simulink model "AdvancedRobotics_PA2_Exercise3"  (R2022a)
settings: Solver=VariableStepAuto  StartTime=0.0  StopTime=10  RelTol=1e-3
values from neighbouring files (symbols this model uses):
  C = CM+CL/n^2    (= 0.0001425)    [AdvancedRobotics_PA2_Exercise3.m]    (also in ControlSystem_transfer_function_ztransform.m = [0 1]; MechDesign_Exercise3_Assessment1.m = k1-(k2+1)*cos(theta_2/180*pi)+k3; PIDTurner.m = pid(Kp,0,Kd); TransferfunctionStateSpace.m = [1 0])
  g = sind(TH2).*sind(TH4) - cosd(TH2).*cosd(TH3).*cosd(TH4)    [AdvancedRobotics_PA2_Exercise2_Group.m]    (also in AdvancedRobotics_PA2_Exercise3.m = 386.1; DigitalFundamental_Lab1_Group.m = 9.8; DigitalFundamental_individual_project_milestone.m = oz*28.3495)
  J = JM+JL/n^2    (= 0.008465)    [AdvancedRobotics_PA2_Exercise3.m]    (also in TransferfunctionStateSpace.m = 0.01)
  Ka = 12    [AdvancedRobotics_PA2_Exercise3.m]
  Kb = 0.00867    [AdvancedRobotics_PA2_Exercise3.m]
  Ke = 1    [AdvancedRobotics_PA2_Exercise3.m]
  KM = 4.375    [AdvancedRobotics_PA2_Exercise3.m]
  L = 0.278    [AdvancedRobotics_PA2_Exercise1_Group.m]    (also in AdvancedRobotics_PA2_Exercise3.m = 0.0006; TransferfunctionStateSpace.m = 0.5)
  l = 6.4    [AdvancedRobotics_PA2_Exercise3.m]
  m = 200    [AdvancedRobotics_PA2_Exercise3.m]    (also in ControlSystem_transfer_function_ztransform.m = 1; DigitalFundamental_individual_project_milestone.m = ft*0.3048)
  n = 200    [AdvancedRobotics_PA2_Exercise3.m]
  R = 1.4    [AdvancedRobotics_PA2_Exercise3.m]    (also in TransferfunctionStateSpace.m = 1)
libraries: simulink x4, slpidlib x2
settings Model: Creator=Thanh  LastModifiedBy=Thanh

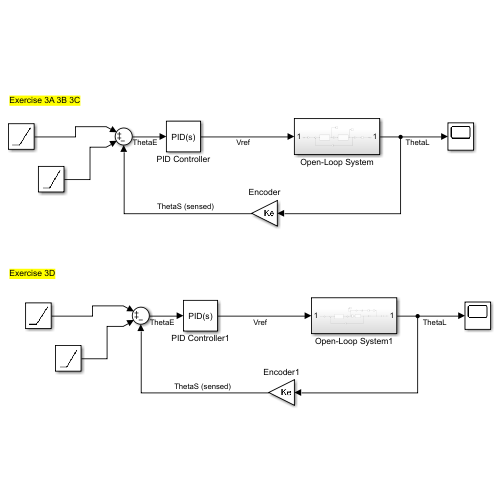
[thumbnail: Simulink's stored preview of the top-level diagram]
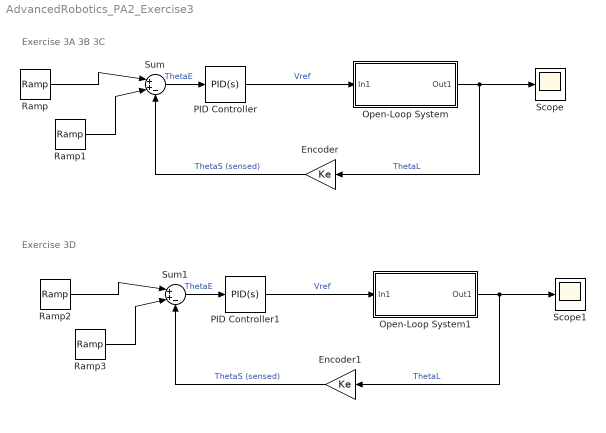
== system AdvancedRobotics_PA2_Exercise3 ==
  note: Exercise 3D
  note: Exercise 3A 3B 3C
  Encoder : Gain  Gain=Ke
  Encoder1 : Gain  Gain=Ke
  Open-Loop System : Subsystem
  Open-Loop System1 : Subsystem
  PID Controller : slpidlib/PID Controller  Controller=PID  Form=Parallel  TimeDomain=Continuous-time  UseExternalTs=off  SampleTime=-1  IntegratorMethod=Forward Euler  FilterMethod=Forward Euler  ControllerParametersSource=internal  P=3.93142383179375  I=1.32077543733285  UseKiTs=off  D=2.60010998792399  N=6581.10544930307  UseFilter=on  TunerSelectOption=Transfer Function Based (PID Tuner App)  InitialConditionSource=internal  InitialConditionForIntegrator=0  InitialConditionForFilter=0  DifferentiatorICPrevScaledInput=0  ExternalReset=none  TrackingMode=off  Kt=1  LimitOutput=off  SatLimitsSource=internal  UpperSaturationLimit=inf  LowerSaturationLimit=-inf  LinearizeAsGain=on  AntiWindupMode=none  Kb=1  POutMin=[]  POutMax=[]  IOutMin=[]  IOutMax=[]  DOutMin=[]  DOutMax=[]  NOutMin=[]  NOutMax=[]  SumOutMin=[]  SumOutMax=[]  SaturationOutMin=[]  SaturationOutMax=[]  PParamMin=[]  PParamMax=[]  IParamMin=[]  IParamMax=[]  DParamMin=[]  DParamMax=[]  NParamMin=[]  NParamMax=[]  KbParamMin=[]  KbParamMax=[]  KtParamMin=[]  KtParamMax=[]  KbOutMin=[]  KbOutMax=[]  KtOutMin=[]  KtOutMax=[]  IntegratorOutMin=[]  IntegratorOutMax=[]  FilterOutMin=[]  FilterOutMax=[]  SumI1OutMin=[]  SumI1OutMax=[]  SumI2OutMin=[]  SumI2OutMax=[]  SumI3OutMin=[]  SumI3OutMax=[]  SumI4OutMin=[]  SumI4OutMax=[]  SumDOutMin=[]  SumDOutMax=[]  DifferentiatorOutMin=[]  DifferentiatorOutMax=[]  FilterDiffOutCoefMin=[]  FilterDiffOutCoefMax=[]  ReciprocalOutMin=[]  ReciprocalOutMax=[]  SumDenOutMin=[]  SumDenOutMax=[]  SumNumOutMin=[]  SumNumOutMax=[]  DivideOutMin=[]  DivideOutMax=[]  UdiffTsProdOutMin=[]  UdiffTsProdOutMax=[]  NTsProdOutMin=[]  NTsProdOutMax=[]  UintegralTsProdOutMin=[]  UintegralTsProdOutMax=[]  UngainTsProdOutMin=[]  UngainTsProdOutMax=[]  IntegratorContinuousStateAttributes=''  IntegratorStateMustResolveToSignalObject=off  IntegratorRTWStateStorageClass=Auto  FilterContinuousStateAttributes=''  FilterStateMustResolveToSignalObject=off  FilterRTWStateStorageClass=Auto  ParallelPVariant=InternalParameters  IdealPVariant=Disabled  IVariant=InternalParameters  DVariant=InternalParameters  IntegratorVariant=Continuous  SatVariant=Disabled  AWVariant=Passthrough  PCopyVariant=Disabled  TRVariant=Disabled  FdbkBlocksVariant=Forward  IdealPFdbkVariant=Disabled  SatFdbkVariant=Disabled  DerivativeFilterVariant=ContFilter  NVariant=InternalParameters  NCopyVariant=Disabled  FilterICVariant=InternalICsFilter  IntegratorICVariant=InternalICs  ExternalResetVariant=Disabled  TRSumVariant=Passthrough  SumFdbkVariant=Disabled  SumVariant=Sum_PID  TsampFilterVariant=InternalTs  TsampNgainVariant=Passthrough  TsampIntegralVariant=Passthrough  ExternalSaturationOutDataTypeStr=Inherit: Same as second input  aMode=0
  PID Controller1 : slpidlib/PID Controller  Controller=PID  Form=Parallel  TimeDomain=Continuous-time  UseExternalTs=off  SampleTime=-1  IntegratorMethod=Forward Euler  FilterMethod=Forward Euler  ControllerParametersSource=internal  P=673.021615306748  I=2889.57947958597  UseKiTs=off  D=34.8292683962231  N=84105.6872201568  UseFilter=on  TunerSelectOption=Transfer Function Based (PID Tuner App)  InitialConditionSource=internal  InitialConditionForIntegrator=0  InitialConditionForFilter=0  DifferentiatorICPrevScaledInput=0  ExternalReset=none  TrackingMode=off  Kt=1  LimitOutput=off  SatLimitsSource=internal  UpperSaturationLimit=inf  LowerSaturationLimit=-inf  LinearizeAsGain=on  AntiWindupMode=none  Kb=1  POutMin=[]  POutMax=[]  IOutMin=[]  IOutMax=[]  DOutMin=[]  DOutMax=[]  NOutMin=[]  NOutMax=[]  SumOutMin=[]  SumOutMax=[]  SaturationOutMin=[]  SaturationOutMax=[]  PParamMin=[]  PParamMax=[]  IParamMin=[]  IParamMax=[]  DParamMin=[]  DParamMax=[]  NParamMin=[]  NParamMax=[]  KbParamMin=[]  KbParamMax=[]  KtParamMin=[]  KtParamMax=[]  KbOutMin=[]  KbOutMax=[]  KtOutMin=[]  KtOutMax=[]  IntegratorOutMin=[]  IntegratorOutMax=[]  FilterOutMin=[]  FilterOutMax=[]  SumI1OutMin=[]  SumI1OutMax=[]  SumI2OutMin=[]  SumI2OutMax=[]  SumI3OutMin=[]  SumI3OutMax=[]  SumI4OutMin=[]  SumI4OutMax=[]  SumDOutMin=[]  SumDOutMax=[]  DifferentiatorOutMin=[]  DifferentiatorOutMax=[]  FilterDiffOutCoefMin=[]  FilterDiffOutCoefMax=[]  ReciprocalOutMin=[]  ReciprocalOutMax=[]  SumDenOutMin=[]  SumDenOutMax=[]  SumNumOutMin=[]  SumNumOutMax=[]  DivideOutMin=[]  DivideOutMax=[]  UdiffTsProdOutMin=[]  UdiffTsProdOutMax=[]  NTsProdOutMin=[]  NTsProdOutMax=[]  UintegralTsProdOutMin=[]  UintegralTsProdOutMax=[]  UngainTsProdOutMin=[]  UngainTsProdOutMax=[]  IntegratorContinuousStateAttributes=''  IntegratorStateMustResolveToSignalObject=off  IntegratorRTWStateStorageClass=Auto  FilterContinuousStateAttributes=''  FilterStateMustResolveToSignalObject=off  FilterRTWStateStorageClass=Auto  ParallelPVariant=InternalParameters  IdealPVariant=Disabled  IVariant=InternalParameters  DVariant=InternalParameters  IntegratorVariant=Continuous  SatVariant=Disabled  AWVariant=Passthrough  PCopyVariant=Disabled  TRVariant=Disabled  FdbkBlocksVariant=Forward  IdealPFdbkVariant=Disabled  SatFdbkVariant=Disabled  DerivativeFilterVariant=ContFilter  NVariant=InternalParameters  NCopyVariant=Disabled  FilterICVariant=InternalICsFilter  IntegratorICVariant=InternalICs  ExternalResetVariant=Disabled  TRSumVariant=Passthrough  SumFdbkVariant=Disabled  SumVariant=Sum_PID  TsampFilterVariant=InternalTs  TsampNgainVariant=Passthrough  TsampIntegralVariant=Passthrough  ExternalSaturationOutDataTypeStr=Inherit: Same as second input  aMode=0
  Ramp : simulink/Sources/Ramp  slope=40  start=0  InitialOutput=0
  Ramp1 : simulink/Sources/Ramp  slope=-40  start=1.5  InitialOutput=0
  Ramp2 : simulink/Sources/Ramp  slope=40  start=0  InitialOutput=0
  Ramp3 : simulink/Sources/Ramp  slope=-40  start=1.5  InitialOutput=0
  Scope : Scope
  Scope1 : Scope
  Sum : Sum  Inputs=|++-
  Sum1 : Sum  Inputs=|++-
  wires:
  PID Controller/1 -> Open-Loop System/1(In1)  "Vref"
  Sum/1 -> PID Controller/1  "ThetaE"
  Encoder/1 -> Sum/3  "ThetaS (sensed)"
  Open-Loop System/1(Out1) -> Scope/1, Encoder/1  "ThetaL"
  Ramp/1 -> Sum/1
  Ramp1/1 -> Sum/2
  Sum1/1 -> PID Controller1/1  "ThetaE"
  Ramp3/1 -> Sum1/2
  PID Controller1/1 -> Open-Loop System1/1(In1)  "Vref"
  Encoder1/1 -> Sum1/3  "ThetaS (sensed)"
  Open-Loop System1/1(Out1) -> Scope1/1, Encoder1/1  "ThetaL"
  Ramp2/1 -> Sum1/1

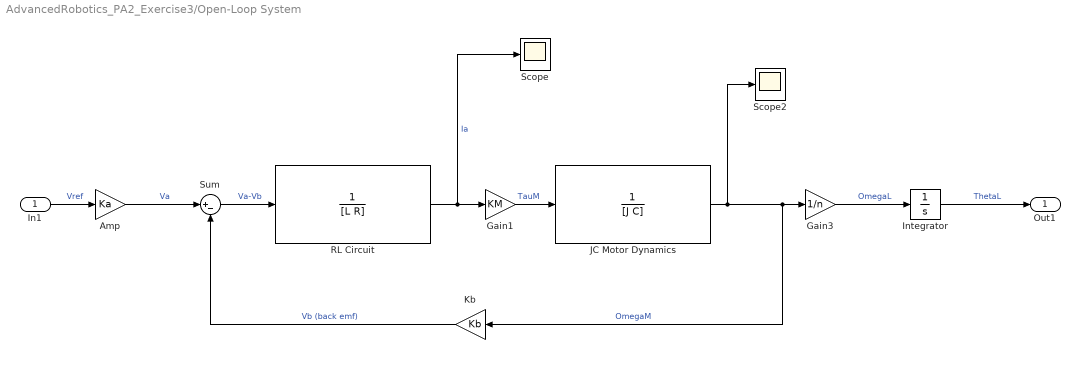
== system AdvancedRobotics_PA2_Exercise3/Open-Loop System ==
  In1 : Inport
  Amp : Gain  Gain=Ka
  Gain1 : Gain  Gain=KM
  Gain3 : Gain  Gain=1/n
  Integrator : Integrator
  JC Motor Dynamics : TransferFcn  Denominator=[J C]
  Kb : Gain  Gain=Kb
  RL Circuit : TransferFcn  Denominator=[L R]
  Scope : Scope
  Scope2 : Scope
  Sum : Sum  Inputs=|+-
  Out1 : Outport
  wires:
  In1/1 -> Amp/1  "Vref"
  Amp/1 -> Sum/1  "Va"
  Kb/1 -> Sum/2  "Vb (back emf)"
  Sum/1 -> RL Circuit/1  "Va-Vb"
  RL Circuit/1 -> Scope/1, Gain1/1  "Ia"
  Gain1/1 -> JC Motor Dynamics/1  "TauM"
  JC Motor Dynamics/1 -> Scope2/1, Kb/1, Gain3/1  "OmegaM"
  Integrator/1 -> Out1/1  "ThetaL"
  Gain3/1 -> Integrator/1  "OmegaL"

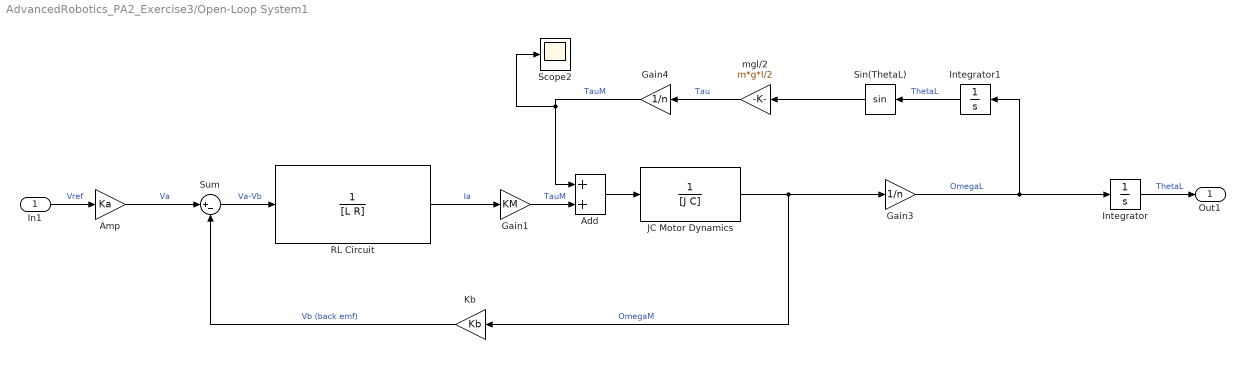
== system AdvancedRobotics_PA2_Exercise3/Open-Loop System1 ==
  In1 : Inport
  Add : Sum
  Amp : Gain  Gain=Ka
  Gain1 : Gain  Gain=KM
  Gain3 : Gain  Gain=1/n
  Gain4 : Gain  Gain=1/n
  Integrator : Integrator
  Integrator1 : Integrator
  JC Motor Dynamics : TransferFcn  Denominator=[J C]
  Kb : Gain  Gain=Kb
  RL Circuit : TransferFcn  Denominator=[L R]
  Scope2 : Scope
  Sin(ThetaL) : Trigonometry
  Sum : Sum  Inputs=|+-
  mgl/2 : Gain  Gain=m*g*l/2
  Out1 : Outport
  wires:
  In1/1 -> Amp/1  "Vref"
  Amp/1 -> Sum/1  "Va"
  Kb/1 -> Sum/2  "Vb (back emf)"
  Sum/1 -> RL Circuit/1  "Va-Vb"
  RL Circuit/1 -> Gain1/1  "Ia"
  Gain1/1 -> Add/2  "TauM"
  JC Motor Dynamics/1 -> Kb/1, Gain3/1  "OmegaM"
  Add/1 -> JC Motor Dynamics/1
  Gain4/1 -> Scope2/1, Add/1  "TauM"
  mgl/2/1 -> Gain4/1  "Tau"
  Sin(ThetaL)/1 -> mgl/2/1
  Integrator/1 -> Out1/1  "ThetaL"
  Gain3/1 -> Integrator/1, Integrator1/1  "OmegaL"
  Integrator1/1 -> Sin(ThetaL)/1  "ThetaL"
